simulink model "Engine_MILS_V1"  (R2017a)
settings: Solver=ode23s  StartTime=0.0  StopTime=10.0  RelTol=1e-3
settings Model: Creator=nishito  LastModifiedBy=nishito

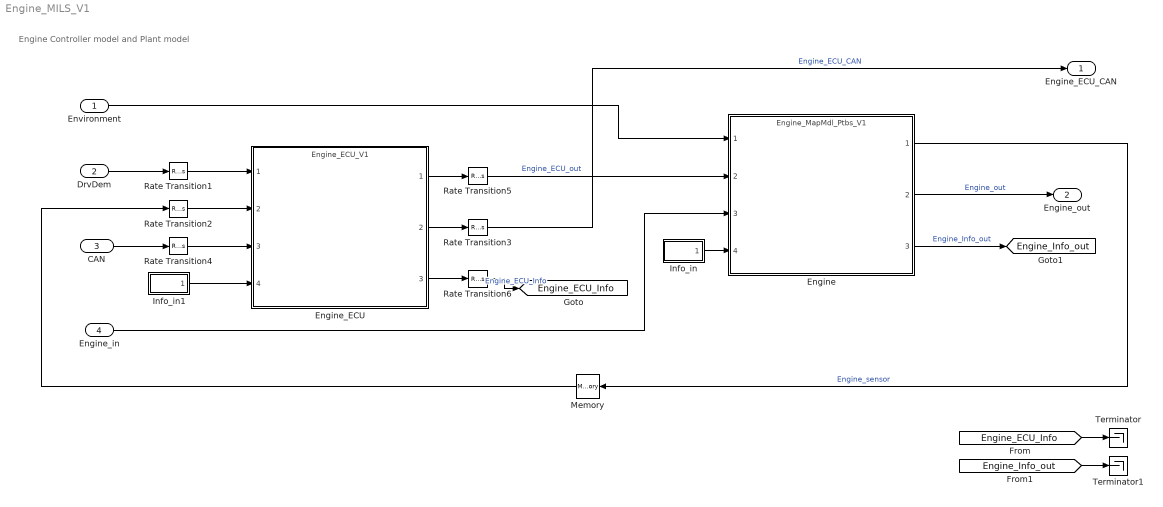
== system Engine_MILS_V1 ==
  note: Engine Controller model and Plant model
  Environment : Inport  OutDataTypeStr=Bus: Environment_Bus
  DrvDem : Inport  Port=2  OutDataTypeStr=Bus: Driver_demand_Bus
  CAN : Inport  Port=3  OutDataTypeStr=Bus: CAN_Bus
  Engine_in : Inport  Port=4  OutDataTypeStr=Bus: Engine_in_Bus
  Engine : ModelReference  ModelNameDialog=Engine_MapMdl_Ptbs_V1.slx  SimulationMode=Normal  ModelReferenceVersion=1.1329
  Engine_ECU : ModelReference  ModelNameDialog=Engine_ECU_V1  SimulationMode=Normal  VariantControl=Variant  ModelReferenceVersion=1.0.6
  Info_in : Subsystem
  Info_in1 : Subsystem
  Memory : Memory
  Rate Transition{1..6} (6 alike) : RateTransition  Deterministic=off
  Terminator : Terminator
  Terminator1 : Terminator
  Engine_ECU_CAN : Outport
  Engine_out : Outport  Port=2  OutDataTypeStr=Bus: Engine_out_Bus
  tag scope: Engine_ECU_Info=global, Engine_Info_out=global
  wires:
  DrvDem/1 -> Rate Transition1/1
  CAN/1 -> Rate Transition4/1
  Engine_ECU/1 -> Rate Transition5/1
  Rate Transition1/1 -> Engine_ECU/1
  Rate Transition4/1 -> Engine_ECU/3
  Engine_ECU/2 -> Rate Transition3/1
  Rate Transition6/1 -> [Engine_ECU_Info]  "Engine_ECU_Info"
  Rate Transition3/1 -> Engine_ECU_CAN/1  "Engine_ECU_CAN"
  Rate Transition2/1 -> Engine_ECU/2
  [Engine_ECU_Info] -> Terminator/1
  [Engine_Info_out] -> Terminator1/1
  Engine/3 -> [Engine_Info_out]  "Engine_Info_out"
  Environment/1 -> Engine/1
  Info_in/1(Info_in) -> Engine/4
  Rate Transition5/1 -> Engine/2  "Engine_ECU_out"
  Engine_in/1 -> Engine/3
  Engine/1 -> Memory/1  "Engine_sensor"
  Memory/1 -> Rate Transition2/1
  Info_in1/1(Info_in) -> Engine_ECU/4
  Engine_ECU/3 -> Rate Transition6/1
  Engine/2 -> Engine_out/1  "Engine_out"

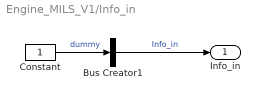
== system Engine_MILS_V1/Info_in ==
  Bus Creator1 : BusCreator  Inputs=1
  Constant : Constant
  Info_in : Outport
  wires:
  Constant/1 -> Bus Creator1/1  "dummy"
  Bus Creator1/1 -> Info_in/1  "Info_in"

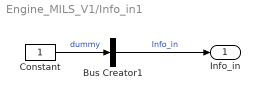
== system Engine_MILS_V1/Info_in1 ==
  Bus Creator1 : BusCreator  Inputs=1
  Constant : Constant
  Info_in : Outport
  wires:
  Bus Creator1/1 -> Info_in/1  "Info_in"
  Constant/1 -> Bus Creator1/1  "dummy"
